simulink model "AutopilotControlSystem"  (R2021b)
settings: configuration reference "ctrlConfigSet" (kept outside this file)
undefined symbols (not defined in the file): ap, DiscIntNeverNeededParam, Earth, env, sensors, uavData, WGS84
libraries: mbdriLib x29, simulink x9, aerolibatmos2 x2, slpidlib x1, simulink_need_slupdate x1, aerolibconvert2 x1, aerolibtransform2 x1
(part 2 of 2)

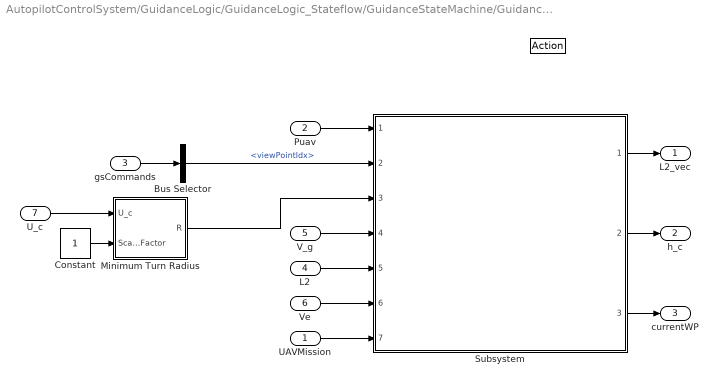
== system AutopilotControlSystem/GuidanceLogic/GuidanceLogic_Stateflow/GuidanceStateMachine/GuidanceLogic.Orbit ==
  UAVMission : Inport
  Puav : Inport  Port=2
  gsCommands : Inport  Port=3
  L2 : Inport  Port=4
  V_g : Inport  Port=5
  Ve : Inport  Port=6
  U_c : Inport  Port=7
  " " : ActionPort
      settings: CopyFcn=Stateflow.SLINSF.SimulinkMan.removeBlockPreDeleteFcn  PreDeleteFcn=Stateflow.SLINSF.SimulinkMan.unsafePredeleteFcn
  Bus Selector : BusSelector  OutputSignals=viewPointIdx
  Constant : Constant  OutDataTypeStr=single
      settings: AttributesFormatString=%<Value>
  Minimum Turn Radius : Subsystem
  Subsystem : Subsystem  ReferencedSubsystem=Orbit
  L2_vec : Outport  VectorParamsAs1DForOutWhenUnconnected=off
  h_c : Outport  Port=2  VectorParamsAs1DForOutWhenUnconnected=off
  currentWP : Outport  Port=3  VectorParamsAs1DForOutWhenUnconnected=off
  wires:
  Subsystem/2 -> h_c/1
  Subsystem/3 -> currentWP/1
  Subsystem/1 -> L2_vec/1
  UAVMission/1 -> Subsystem/7
  Puav/1 -> Subsystem/1
  gsCommands/1 -> Bus Selector/1
  Bus Selector/1 -> Subsystem/2  "<viewPointIdx>"
  Constant/1 -> Minimum Turn Radius/2(Scale Factor)
  U_c/1 -> Minimum Turn Radius/1(U_c)
  Minimum Turn Radius/1(R) -> Subsystem/3
  L2/1 -> Subsystem/5
  V_g/1 -> Subsystem/4
  Ve/1 -> Subsystem/6

== system AutopilotControlSystem/GuidanceLogic/GuidanceLogic_Stateflow/GuidanceStateMachine/GuidanceLogic.RTB ==
  gsCommands : Inport  OutDataTypeStr=Bus: gsCommandsBus
  UAVMission : Inport  Port=2
  Puav : Inport  Port=3
  " " : ActionPort
      settings: CopyFcn=Stateflow.SLINSF.SimulinkMan.removeBlockPreDeleteFcn  PreDeleteFcn=Stateflow.SLINSF.SimulinkMan.unsafePredeleteFcn
  Bus Selector : BusSelector  OutputSignals=MobileLocation,followMobile,h_c_midLevel
  Subsystem : Subsystem  ReferencedSubsystem=RTB_FollowMobile
  L2_vec : Outport  VectorParamsAs1DForOutWhenUnconnected=off
  h_c : Outport  Port=2  VectorParamsAs1DForOutWhenUnconnected=off
  currentWP : Outport  Port=3  VectorParamsAs1DForOutWhenUnconnected=off
  wires:
  Subsystem/2 -> h_c/1
  Subsystem/1 -> L2_vec/1
  Subsystem/3 -> currentWP/1
  Puav/1 -> Subsystem/4
  UAVMission/1 -> Subsystem/5
  gsCommands/1 -> Bus Selector/1
  Bus Selector/1 -> Subsystem/1  "<MobileLocation>"
  Bus Selector/2 -> Subsystem/2  "<followMobile>"
  Bus Selector/3 -> Subsystem/3  "<h_c_midLevel>"

== system AutopilotControlSystem/GuidanceLogic/GuidanceLogic_Stateflow/GuidanceStateMachine/GuidanceLogic.WP ==
  apConfigParams : Inport
  UAVMission : Inport  Port=2
  Puav : Inport  Port=3
  L2 : Inport  Port=4
  V_g : Inport  Port=5
  wpEnable : Inport  Port=6
  " " : ActionPort
      settings: CopyFcn=Stateflow.SLINSF.SimulinkMan.removeBlockPreDeleteFcn  PreDeleteFcn=Stateflow.SLINSF.SimulinkMan.unsafePredeleteFcn
  Bus Selector : BusSelector  OutputSignals=turnLead
  MATLAB Function : MATLAB Function  TreatAsAtomicUnit=on
  Subsystem Reference : Subsystem  ReferencedSubsystem=WP_Guidance
  L2_vec : Outport  VectorParamsAs1DForOutWhenUnconnected=off
  h_c : Outport  Port=2  VectorParamsAs1DForOutWhenUnconnected=off
  currentWP : Outport  Port=3  VectorParamsAs1DForOutWhenUnconnected=off
  wires:
  UAVMission/1 -> MATLAB Function/1(u), Subsystem Reference/1
  Subsystem Reference/3 -> currentWP/1
  Subsystem Reference/2 -> h_c/1
  Subsystem Reference/1 -> L2_vec/1
  Puav/1 -> Subsystem Reference/2
  L2/1 -> Subsystem Reference/3
  MATLAB Function/1(maxWp) -> Subsystem Reference/4
  apConfigParams/1 -> Bus Selector/1
  Bus Selector/1 -> Subsystem Reference/5  "<turnLead>"
  V_g/1 -> Subsystem Reference/6
  wpEnable/1 -> Subsystem Reference/7

== system AutopilotControlSystem/GuidanceLogic/GuidanceLogic_Stateflow/Recent Enable ==
  WP Fly : Inport
  IC1 : InitialCondition  Value=0
  Subsystem : Subsystem
  WPEnable : Outport  VectorParamsAs1DForOutWhenUnconnected=off
  wires:
  WP Fly/1 -> IC1/1
  Subsystem/1(Just Enab) -> WPEnable/1
  IC1/1 -> Subsystem/1(WP Fly)

== system AutopilotControlSystem/InnerLoopAutopilot/Latch Trim Conditions/Latch Control Surfaces Trim from any mode ==
  ctrlSurfaces : Inport
  Trigger : TriggerPort  TriggerType=falling  VariantControl=Variant
  Trim : Outport  VectorParamsAs1DForOutWhenUnconnected=off
  wires:
  ctrlSurfaces/1 -> Trim/1

== system AutopilotControlSystem/InnerLoopAutopilot/Longitudinal Channel/Compute Feed Forward ==
  dEFFGain : Inport
  SensorData : Inport  Port=2
  1D Discrete Filter : mbdriLib/Filtering/1D Discrete Filter  bw=10  TSample=ap.apSampleTime
      settings: AttributesFormatString=Fc = 10
  Add5 : Sum  Inputs=+-  OutDataTypeStr=single
  Bus Selector : BusSelector  OutputSignals=Euler
  Constant2 : Constant  OutDataTypeStr=single
      settings: AttributesFormatString=%<Value>
  Constant4 : Constant  OutDataTypeStr=single
      settings: AttributesFormatString=%<Value>
  Product : Product  Inputs=*/  RndMeth=Zero
  Product1 : Product  RndMeth=Zero
  Selector : Selector  InputPortWidth=3  IndexOptions=Index vector (dialog)  Indices=[1]  OutputSizes=1
  Trigonometric Function : Trigonometry  Operator=cos
  "[-60 60]" : Saturate  UpperLimit=60  LowerLimit=-60
      settings: AttributesFormatString="[%<LowerLimit>  %<UpperLimit>]"
  FF : Outport  VectorParamsAs1DForOutWhenUnconnected=off
  wires:
  Selector/1 -> 1D Discrete Filter/1
  Product/1 -> Add5/1
  Constant4/1 -> Product/1
  1D Discrete Filter/1 -> "[-60 60]"/1
  Trigonometric Function/1 -> Product/2
  Constant2/1 -> Add5/2
  Product1/1 -> FF/1
  Add5/1 -> Product1/2
  "[-60 60]"/1 -> Trigonometric Function/1
  Bus Selector/1 -> Selector/1  "<Euler>"
  dEFFGain/1 -> Product1/1
  SensorData/1 -> Bus Selector/1

== system AutopilotControlSystem/InnerLoopAutopilot/Longitudinal Channel/Height Error to Pitch Command [PI] ==
  Error : Inport
  Reset : Inport  Port=2
  PIDGains : Inport  Port=3
  Cast To Boolean : DataTypeConversion  OutDataTypeStr=boolean
  Demux : Demux  Outputs=3
  PID Controller : slpidlib/PID Controller  Controller=PI  Form=Parallel  TimeDomain=Discrete-time  UseExternalTs=off  SampleTime=ap.apSampleTime  IntegratorMethod=Trapezoidal  FilterMethod=Forward Euler  ControllerParametersSource=external  P=1  I=1  D=0  UseFilter=on  N=100  TunerSelectOption=Transfer Function Based (PID Tuner App)  InitialConditionSource=internal  InitialConditionForIntegrator=0  InitialConditionForFilter=0  DifferentiatorICPrevScaledInput=0  ExternalReset=level  TrackingMode=off  Kt=1  LimitOutput=on  SatLimitsSource=internal  UpperSaturationLimit=ap.control.the_cLimit  LowerSaturationLimit=-ap.control.the_cLimit  LinearizeAsGain=on  AntiWindupMode=clamping  Kb=1  POutMin=[]  POutMax=[]  IOutMin=[]  IOutMax=[]  DOutMin=[]  DOutMax=[]  NOutMin=[]  NOutMax=[]  SumOutMin=[]  SumOutMax=[]  SaturationOutMin=[]  SaturationOutMax=[]  PParamMin=[]  PParamMax=[]  IParamMin=[]  IParamMax=[]  DParamMin=[]  DParamMax=[]  NParamMin=[]  NParamMax=[]  KbParamMin=[]  KbParamMax=[]  KtParamMin=[]  KtParamMax=[]  KbOutMin=[]  KbOutMax=[]  KtOutMin=[]  KtOutMax=[]  IntegratorOutMin=[]  IntegratorOutMax=[]  FilterOutMin=[]  FilterOutMax=[]  SumI1OutMin=[]  SumI1OutMax=[]  SumI2OutMin=[]  SumI2OutMax=[]  SumI3OutMin=[]  SumI3OutMax=[]  SumI4OutMin=[]  SumI4OutMax=[]  SumDOutMin=[]  SumDOutMax=[]  DifferentiatorOutMin=[]  DifferentiatorOutMax=[]  FilterDiffOutCoefMin=[]  FilterDiffOutCoefMax=[]  ReciprocalOutMin=[]  ReciprocalOutMax=[]  SumDenOutMin=[]  SumDenOutMax=[]  SumNumOutMin=[]  SumNumOutMax=[]  DivideOutMin=[]  DivideOutMax=[]  UdiffTsProdOutMin=[]  UdiffTsProdOutMax=[]  NTsProdOutMin=[]  NTsProdOutMax=[]  UintegralTsProdOutMin=[]  UintegralTsProdOutMax=[]  UngainTsProdOutMin=[]  UngainTsProdOutMax=[]  IntegratorContinuousStateAttributes=''  IntegratorStateMustResolveToSignalObject=off  IntegratorRTWStateStorageClass=Auto  FilterContinuousStateAttributes=''  FilterStateMustResolveToSignalObject=off  FilterRTWStateStorageClass=Auto  ParallelPVariant=ExternalParameters  IdealPVariant=Disabled  IVariant=ExternalParameters  DVariant=Disabled  IntegratorVariant=Discrete  SatVariant=Enabled  AWVariant=DiscClampingParallel  PCopyVariant=Disabled  TRVariant=Disabled  FdbkBlocksVariant=Feedback  IdealPFdbkVariant=Passthrough  SatFdbkVariant=Passthrough  DerivativeFilterVariant=Disabled  NVariant=Disabled  NCopyVariant=Disabled_SignalSpec  FilterICVariant=Disabled  IntegratorICVariant=InternalICs  ExternalResetVariant=ExternalReset  TRSumVariant=Passthrough  SumFdbkVariant=Enabled  SumVariant=Sum_PI  TsampFilterVariant=InternalTs  TsampNgainVariant=Passthrough  TsampIntegralVariant=Passthrough  ExternalSaturationOutDataTypeStr=Inherit: Same as second input
  Terminator : Terminator
  Output : Outport  VectorParamsAs1DForOutWhenUnconnected=off
  wires:
  Demux/3 -> Terminator/1
  Error/1 -> PID Controller/1
  PIDGains/1 -> Demux/1
  Demux/1 -> PID Controller/2
  Demux/2 -> PID Controller/3
  Reset/1 -> Cast To Boolean/1
  PID Controller/1 -> Output/1
  Cast To Boolean/1 -> PID Controller/4

== system AutopilotControlSystem/InnerLoopAutopilot/Longitudinal Channel/Rate Limiter Dynamic with External IC and Autoreset for Change in IC ==
  note: Y(k)
  note: U(k)
  up : Inport
  u : Inport  Port=2
  IC : Inport  Port=3
  lo : Inport  Port=4
  Capture/Reset IC : Subsystem
  Difference Inputs1 : Sum  Description=Add in CPU  DisableCoverage=on  Inputs=+-  OutDataTypeStr=Inherit: Inherit via back propagation
  Difference Inputs2 : Sum  Description=Add in CPU  OutDataTypeStr=Inherit: Inherit via back propagation
  FixPt Data Type Duplicate : DataTypeDuplicate  DisableCoverage=on  NumInputPorts=7
  Saturation Dynamic : simulink/Discontinuities/Saturation Dynamic  OutMin=[]  OutMax=[]  OutDataTypeStr=Inherit: Same as second input  OutDataType=fixdt(1, 16)  OutScaling=2^-10  DoSatur=off
  delta fall limit : Product  DisableCoverage=on  Inputs=**  OutDataTypeStr=Inherit: Inherit via back propagation  SaturateOnIntegerOverflow=on
  delta rise limit : Product  DisableCoverage=on  Inputs=**  OutDataTypeStr=Inherit: Inherit via back propagation  SaturateOnIntegerOverflow=on
  sample time : SampleTimeMath  DisableCoverage=on  TsampMathOp=Ts Only  weightValue=1
  Y : Outport  VectorParamsAs1DForOutWhenUnconnected=off
  wires:
  sample time/1 -> delta fall limit/2, delta rise limit/2
  lo/1 -> delta fall limit/1
  delta rise limit/1 -> FixPt Data Type Duplicate/6, Saturation Dynamic/1
  up/1 -> delta rise limit/1
  Difference Inputs2/1 -> FixPt Data Type Duplicate/1, Capture/Reset IC/1(Y(k)), Y/1
  Saturation Dynamic/1 -> Difference Inputs2/1, FixPt Data Type Duplicate/7
  delta fall limit/1 -> FixPt Data Type Duplicate/3, Saturation Dynamic/3
  u/1 -> Difference Inputs1/1, FixPt Data Type Duplicate/5, sample time/1
  Difference Inputs1/1 -> FixPt Data Type Duplicate/4, Saturation Dynamic/2  "( U(k) - Y(k-1) )"
  Capture/Reset IC/1(Y(k-1)) -> Difference Inputs2/2, FixPt Data Type Duplicate/2, Difference Inputs1/2
  IC/1 -> Capture/Reset IC/2(IC)

== system AutopilotControlSystem/Navigation Filter/Get Vn Ve/Subsystem5 ==
  u : Inport
  Trigonometric Function : Trigonometry
  Trigonometric Function1 : Trigonometry  Operator=cos
  sin(u) : Outport  VectorParamsAs1DForOutWhenUnconnected=off
  cos(u) : Outport  Port=2  VectorParamsAs1DForOutWhenUnconnected=off
  wires:
  u/1 -> Trigonometric Function/1, Trigonometric Function1/1
  Trigonometric Function/1 -> sin(u)/1
  Trigonometric Function1/1 -> cos(u)/1

== system AutopilotControlSystem/Navigation Filter/Position&Velocity Filter/CompRateOnly ==
  LoPass : Inport
  Gain : Gain  Gain=omega
      settings: AttributesFormatString=%<Gain>
  Sum1 : Sum  Inputs=|+-
  Unit Delay : UnitDelay  SampleTime=T  HasFrameUpgradeWarning=on
  ZPK 1D Discrete Filter : mbdriLib/Filtering/ZPK 1D Discrete Filter  zval=[]  pval=[0]  kval=1  TSample=0.01
  Rate_hat : Outport  VectorParamsAs1DForOutWhenUnconnected=off
  wires:
  Unit Delay/1 -> Sum1/2
  LoPass/1 -> Sum1/1
  Sum1/1 -> Gain/1
  Gain/1 -> ZPK 1D Discrete Filter/1, Rate_hat/1
  ZPK 1D Discrete Filter/1 -> Unit Delay/1

== system AutopilotControlSystem/Navigation Filter/Position&Velocity Filter/Deriv  ==
  y : Inport
  Gain2 : Gain  Gain=[ 1/(5*ap.apSampleTime) ]
      settings: AttributesFormatString=%<Gain>
  Integer Delay1 : Delay  DelayLength=5  InitialCondition=0
  Sum5 : Sum  Inputs=-+|
  ydot : Outport  VectorParamsAs1DForOutWhenUnconnected=off
  wires:
  Gain2/1 -> ydot/1
  y/1 -> Integer Delay1/1, Sum5/2
  Integer Delay1/1 -> Sum5/1
  Sum5/1 -> Gain2/1

== system AutopilotControlSystem/Navigation Filter/Position&Velocity Filter/VN Ve Filter ==
  Vn : Inport
  Ve : Inport  Port=2
  New GPS : Inport  Port=3
  Enable : EnablePort
  Constant : Constant  Value=ap.apSampleTime
      settings: AttributesFormatString=%<Value>
  RateAid for GPS : mbdriLib/Filtering/RateAid for GPS  SystemSampleTime=-1  VariantActivationTime=update diagram  Latency=0  AutoFrameSizeCalculation=off
  RateAid for GPS1 : mbdriLib/Filtering/RateAid for GPS  SystemSampleTime=-1  VariantActivationTime=update diagram  Latency=0  AutoFrameSizeCalculation=off
  Vn_fil : Outport  OutputWhenDisabled=reset  InitialOutput=0  VectorParamsAs1DForOutWhenUnconnected=off
  Ve_fil : Outport  Port=2  OutputWhenDisabled=reset  InitialOutput=0  VectorParamsAs1DForOutWhenUnconnected=off
  wires:
  Constant/1 -> RateAid for GPS1/3, RateAid for GPS/3
  New GPS/1 -> RateAid for GPS/2, RateAid for GPS1/2
  Vn/1 -> RateAid for GPS/1
  Ve/1 -> RateAid for GPS1/1
  RateAid for GPS/1 -> Vn_fil/1
  RateAid for GPS1/1 -> Ve_fil/1

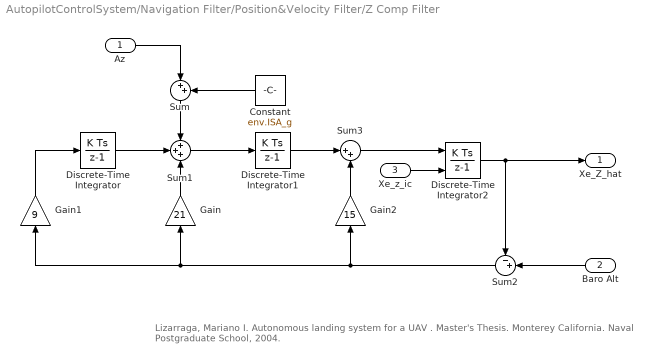
== system AutopilotControlSystem/Navigation Filter/Position&Velocity Filter/Z Comp Filter ==
  note: Lizarraga, Mariano I. Autonomous landing system for a UAV . Master's Thesis. Monterey California. Naval Postgraduate School, 2004.
  Az : Inport
  Baro Alt : Inport  Port=2
  Xe_z_ic : Inport  Port=3
  Constant : Constant  Value=env.ISA_g
      settings: AttributesFormatString=%<Value>
  Discrete-Time Integrator : DiscreteIntegrator  gainval=1  SampleTime=-1  ICPrevOutput=DiscIntNeverNeededParam  ICPrevScaledInput=DiscIntNeverNeededParam
  Discrete-Time Integrator1 : DiscreteIntegrator  gainval=1  SampleTime=-1  ICPrevOutput=DiscIntNeverNeededParam  ICPrevScaledInput=DiscIntNeverNeededParam
  Discrete-Time Integrator2 : DiscreteIntegrator  gainval=1  InitialConditionSource=external  SampleTime=-1  ICPrevOutput=DiscIntNeverNeededParam  ICPrevScaledInput=DiscIntNeverNeededParam
  Gain : Gain  Gain=21  OutDataTypeStr=single
      settings: AttributesFormatString=%<Gain>
  Gain1 : Gain  Gain=9  OutDataTypeStr=single
      settings: AttributesFormatString=%<Gain>
  Gain2 : Gain  Gain=15  OutDataTypeStr=single
      settings: AttributesFormatString=%<Gain>
  Sum : Sum  Inputs=|++
  Sum1 : Sum  Inputs=+++
  Sum2 : Sum  Inputs=-+|
  Sum3 : Sum  Inputs=|++
  Xe_Z_hat : Outport  VectorParamsAs1DForOutWhenUnconnected=off
  wires:
  Discrete-Time Integrator2/1 -> Sum2/1, Xe_Z_hat/1
  Gain2/1 -> Sum3/2
  Gain1/1 -> Discrete-Time Integrator/1
  Gain/1 -> Sum1/3
  Sum2/1 -> Gain2/1, Gain/1, Gain1/1
  Sum3/1 -> Discrete-Time Integrator2/1
  Discrete-Time Integrator1/1 -> Sum3/1
  Baro Alt/1 -> Sum2/2
  Xe_z_ic/1 -> Discrete-Time Integrator2/2
  Sum1/1 -> Discrete-Time Integrator1/1
  Sum/1 -> Sum1/1
  Discrete-Time Integrator/1 -> Sum1/2
  Constant/1 -> Sum/2
  Az/1 -> Sum/1

== system AutopilotControlSystem/GuidanceLogic/GuidanceLogic_Simulink/Determine RTB/getHeartbeatAge ==
  Heartbeat : Inport
  Constant : Constant
  Discrete-Time Integrator : DiscreteIntegrator  ExternalReset=level  SampleTime=-1  LimitOutput=on  UpperSaturationLimit=50  LowerSaturationLimit=0  ICPrevOutput=DiscIntNeverNeededParam  ICPrevScaledInput=DiscIntNeverNeededParam
  Age : Outport  VectorParamsAs1DForOutWhenUnconnected=off
  wires:
  Heartbeat/1 -> Discrete-Time Integrator/2
  Discrete-Time Integrator/1 -> Age/1
  Constant/1 -> Discrete-Time Integrator/1

== system AutopilotControlSystem/GuidanceLogic/GuidanceLogic_Simulink/Guidance/Circle Guidance ==
  Xe : Inport
  InterestPoint : Inport  Port=2
  R : Inport  Port=3
  |V_g| : Inport  Port=4
  L2 : Inport  Port=5
  Ve : Inport  Port=6
  UAVMission : Inport  Port=7
  Action Port : ActionPort  ActionPortLabel=elseif( u1 == 3)
  Subsystem : Subsystem  ReferencedSubsystem=Orbit
  L2_vec : Outport  VectorParamsAs1DForOutWhenUnconnected=off
  h_c : Outport  Port=2  VectorParamsAs1DForOutWhenUnconnected=off
  currentWP : Outport  Port=3  VectorParamsAs1DForOutWhenUnconnected=off
  wires:
  |V_g|/1 -> Subsystem/4
  Subsystem/1 -> L2_vec/1
  Subsystem/3 -> currentWP/1
  Subsystem/2 -> h_c/1
  UAVMission/1 -> Subsystem/7
  Ve/1 -> Subsystem/6
  L2/1 -> Subsystem/5
  R/1 -> Subsystem/3
  InterestPoint/1 -> Subsystem/2
  Xe/1 -> Subsystem/1

== system AutopilotControlSystem/GuidanceLogic/GuidanceLogic_Simulink/Guidance/Mid Level Direct Commands ==
  psiDot_c_ml : Inport
  h_c_midLvl : Inport  Port=2
  U_m : Inport  Port=3
  Action Port : ActionPort  ActionPortLabel=elseif( u1 == 4)
  Subsystem : Subsystem  ReferencedSubsystem=DirectCommands
  phi_c_ml : Outport  VectorParamsAs1DForOutWhenUnconnected=off
  h_c : Outport  Port=2  VectorParamsAs1DForOutWhenUnconnected=off
  currentWP : Outport  Port=3  VectorParamsAs1DForOutWhenUnconnected=off
  wires:
  Subsystem/3 -> currentWP/1
  Subsystem/2 -> h_c/1
  Subsystem/1 -> phi_c_ml/1
  U_m/1 -> Subsystem/3
  psiDot_c_ml/1 -> Subsystem/1
  h_c_midLvl/1 -> Subsystem/2

== system AutopilotControlSystem/GuidanceLogic/GuidanceLogic_Simulink/Guidance/Minimum Turn Radius ==
  U_c : Inport
  Scale Factor : Inport  Port=2
  Constant1 : Constant  Value=ap.guidance.maxAcc
      settings: AttributesFormatString=%<Value>
  IC : InitialCondition  Value=1.5
  Math Function : Math  Operator=square  SignedPower=on  SaturateOnIntegerOverflow=on
  Product2 : Product  RndMeth=Zero
  Product3 : Product  Inputs=*/  RndMeth=Zero
  "[1.5 10]" : Saturate  UpperLimit=10  LowerLimit=1.5
      settings: AttributesFormatString="[%<LowerLimit>  %<UpperLimit>]"
  R : Outport  VectorParamsAs1DForOutWhenUnconnected=off
  wires:
  IC/1 -> "[1.5 10]"/1
  "[1.5 10]"/1 -> Product2/1
  Product3/1 -> R/1
  Scale Factor/1 -> IC/1
  Math Function/1 -> Product2/2
  Constant1/1 -> Product3/2
  Product2/1 -> Product3/1
  U_c/1 -> Math Function/1

== system AutopilotControlSystem/GuidanceLogic/GuidanceLogic_Simulink/Guidance/RTB//Follow Mobile Guidance ==
  Mobile Location : Inport
  Follow Mobile? : Inport  Port=2
  MidLvl h_c : Inport  Port=3
  Puav : Inport  Port=4
  UAVMission : Inport  Port=5
  Action Port : ActionPort  ActionPortLabel=if(u2 == 1)
  Subsystem : Subsystem  ReferencedSubsystem=RTB_FollowMobile
  L2_vec : Outport  VectorParamsAs1DForOutWhenUnconnected=off
  h_c : Outport  Port=2  VectorParamsAs1DForOutWhenUnconnected=off
  currentWP : Outport  Port=3  VectorParamsAs1DForOutWhenUnconnected=off
  wires:
  Mobile Location/1 -> Subsystem/1
  Follow Mobile?/1 -> Subsystem/2
  MidLvl h_c/1 -> Subsystem/3
  Puav/1 -> Subsystem/4
  UAVMission/1 -> Subsystem/5
  Subsystem/1 -> L2_vec/1
  Subsystem/2 -> h_c/1
  Subsystem/3 -> currentWP/1

== system AutopilotControlSystem/GuidanceLogic/GuidanceLogic_Simulink/Guidance/Recent Enable ==
  WP Fly : Inport
  IC1 : InitialCondition  Value=0
  Subsystem : Subsystem
  WPEnable : Outport  VectorParamsAs1DForOutWhenUnconnected=off
  wires:
  WP Fly/1 -> IC1/1
  Subsystem/1(Just Enab) -> WPEnable/1
  IC1/1 -> Subsystem/1(WP Fly)

== system AutopilotControlSystem/GuidanceLogic/GuidanceLogic_Simulink/Guidance/WP Guidance ==
  UAVMission : Inport
  Xe : Inport  Port=2
  L2 : Inport  Port=3
  MaxWP : Inport  Port=4
  turnLeadTime : Inport  Port=5
  V_g : Inport  Port=6
  WpEnable : Inport  Port=7
  Action Port : ActionPort  ActionPortLabel=elseif(u1 == 2)
  Subsystem Reference : Subsystem  ReferencedSubsystem=WP_Guidance
  L2Vec : Outport  VectorParamsAs1DForOutWhenUnconnected=off
  h_c : Outport  Port=2  VectorParamsAs1DForOutWhenUnconnected=off
  currentWP : Outport  Port=3  VectorParamsAs1DForOutWhenUnconnected=off
  wires:
  Subsystem Reference/1 -> L2Vec/1
  Subsystem Reference/2 -> h_c/1
  Subsystem Reference/3 -> currentWP/1
  UAVMission/1 -> Subsystem Reference/1
  Xe/1 -> Subsystem Reference/2
  L2/1 -> Subsystem Reference/3
  MaxWP/1 -> Subsystem Reference/4
  turnLeadTime/1 -> Subsystem Reference/5
  V_g/1 -> Subsystem Reference/6
  WpEnable/1 -> Subsystem Reference/7

== system AutopilotControlSystem/GuidanceLogic/GuidanceLogic_Stateflow/Determine RTB/getHeartbeatAge ==
  Heartbeat : Inport
  Constant : Constant
  Discrete-Time Integrator : DiscreteIntegrator  ExternalReset=level  SampleTime=-1  LimitOutput=on  UpperSaturationLimit=50  LowerSaturationLimit=0  ICPrevOutput=DiscIntNeverNeededParam  ICPrevScaledInput=DiscIntNeverNeededParam
  Age : Outport  VectorParamsAs1DForOutWhenUnconnected=off
  wires:
  Heartbeat/1 -> Discrete-Time Integrator/2
  Discrete-Time Integrator/1 -> Age/1
  Constant/1 -> Discrete-Time Integrator/1

== system AutopilotControlSystem/GuidanceLogic/GuidanceLogic_Stateflow/GuidanceStateMachine/GuidanceLogic.Orbit/Minimum Turn Radius ==
  U_c : Inport
  Scale Factor : Inport  Port=2
  Constant1 : Constant  Value=ap.guidance.maxAcc
      settings: AttributesFormatString=%<Value>
  IC : InitialCondition  Value=1.5
  Math Function : Math  Operator=square  SignedPower=on  SaturateOnIntegerOverflow=on
  Product2 : Product  RndMeth=Zero
  Product3 : Product  Inputs=*/  RndMeth=Zero
  "[1.5 10]" : Saturate  UpperLimit=10  LowerLimit=1.5
      settings: AttributesFormatString="[%<LowerLimit>  %<UpperLimit>]"
  R : Outport  VectorParamsAs1DForOutWhenUnconnected=off
  wires:
  IC/1 -> "[1.5 10]"/1
  "[1.5 10]"/1 -> Product2/1
  Product3/1 -> R/1
  Scale Factor/1 -> IC/1
  Math Function/1 -> Product2/2
  Constant1/1 -> Product3/2
  Product2/1 -> Product3/1
  U_c/1 -> Math Function/1

== system AutopilotControlSystem/GuidanceLogic/GuidanceLogic_Stateflow/Recent Enable/Subsystem ==
  WP Fly : Inport
  Data Type Conversion1 : DataTypeConversion  OutDataTypeStr=double
  Data Type Conversion2 : DataTypeConversion  OutDataTypeStr=uint8
  Hit Crossing : HitCross  HitCrossingOffset=0.5  HitCrossingDirection=rising
  Just Enab : Outport  VectorParamsAs1DForOutWhenUnconnected=off
  wires:
  Data Type Conversion1/1 -> Hit Crossing/1
  Hit Crossing/1 -> Data Type Conversion2/1
  Data Type Conversion2/1 -> Just Enab/1
  WP Fly/1 -> Data Type Conversion1/1

== system AutopilotControlSystem/InnerLoopAutopilot/Longitudinal Channel/Rate Limiter Dynamic with External IC and Autoreset for Change in IC/Capture//Reset IC ==
  Y(k) : Inport
  IC : Inport  Port=2
  Abs : Abs
  Delay : Delay  DelayLength=1
  Subsystem : Subsystem
  Subtract : Sum  Inputs=+-
  Unit Delay Resettable External IC : simulink_need_slupdate/Unit Delay Resettable External IC  tsamp=-1
      settings: SourceProductBaseCode=SL
  Y(k-1) : Outport  VectorParamsAs1DForOutWhenUnconnected=off
  wires:
  Unit Delay Resettable External IC/1 -> Y(k-1)/1  "Y(k-1)"
  Y(k)/1 -> Unit Delay Resettable External IC/1
  Subtract/1 -> Abs/1
  Abs/1 -> Subsystem/1(WP Fly)
  IC/1 -> Delay/1, Subtract/2, Unit Delay Resettable External IC/3
  Subsystem/1(Just Enab) -> Unit Delay Resettable External IC/2
  Delay/1 -> Subtract/1

== system AutopilotControlSystem/GuidanceLogic/GuidanceLogic_Simulink/Guidance/Recent Enable/Subsystem ==
  WP Fly : Inport
  Data Type Conversion1 : DataTypeConversion  OutDataTypeStr=double
  Data Type Conversion2 : DataTypeConversion  OutDataTypeStr=uint8
  Hit Crossing : HitCross  HitCrossingOffset=0.5  HitCrossingDirection=rising
  Just Enab : Outport  VectorParamsAs1DForOutWhenUnconnected=off
  wires:
  Data Type Conversion1/1 -> Hit Crossing/1
  Hit Crossing/1 -> Data Type Conversion2/1
  Data Type Conversion2/1 -> Just Enab/1
  WP Fly/1 -> Data Type Conversion1/1

== system AutopilotControlSystem/InnerLoopAutopilot/Longitudinal Channel/Rate Limiter Dynamic with External IC and Autoreset for Change in IC/Capture//Reset IC/Subsystem ==
  WP Fly : Inport
  Compare To Constant : simulink/Logic and Bit Operations/Compare To Constant  relop=>=  const=0.5  OutDataTypeStr=boolean
  Compare To Constant1 : simulink/Logic and Bit Operations/Compare To Constant  relop=<  const=0.5  OutDataTypeStr=boolean
  Logical Operator : Logic  AllPortsSameDT=off  OutDataTypeStr=boolean
  Unit Delay : UnitDelay  SampleTime=-1  HasFrameUpgradeWarning=on
  Just Enab : Outport  VectorParamsAs1DForOutWhenUnconnected=off
  wires:
  WP Fly/1 -> Unit Delay/1, Compare To Constant/1
  Compare To Constant/1 -> Logical Operator/1
  Compare To Constant1/1 -> Logical Operator/2
  Unit Delay/1 -> Compare To Constant1/1
  Logical Operator/1 -> Just Enab/1

== matlab function AutopilotControlSystem/GuidanceLogic/GuidanceLogic_Stateflow/GuidanceStateMachine/GuidanceLogic.WP/MATLAB Function ==
  data: u input Bus: waypoint size=10; maxWp output
function maxWp = getMaxWp(u)
%#codegen

for ii=1:10
    wp = u(ii);
    if wp.wpPos(1) == 0
        maxWp = uint8(ii-1);
        return 
    end
end

maxWp = uint8(10);

== stateflow chart AutopilotControlSystem/GuidanceLogic/GuidanceLogic_Stateflow/GuidanceStateMachine ==
  settings: updateMethod=DISCRETE  sampleTime=ap.apSampleTime
  state GuidanceLogic
    state RTB
    state WP
    state Orbit
    state MidLevel
    (default) -> (junction 43)
    (junction 83) -> RTB
    (junction 82) -> (junction 83)
    (junction 43) -> RTB [order 1] : [RTB==1]
    (junction 43) -> (junction 19) [order 2]
    (junction 19) -> WP [order 1] : [guidanceMode == 2]
    (junction 19) -> (junction 27) [order 2]
    (junction 27) -> Orbit [order 1] : [guidanceMode == 3]
    (junction 27) -> (junction 32) [order 2]
    (junction 32) -> MidLevel [order 1] : [guidanceMode == 4]
    (junction 32) -> (junction 84) [order 2]
    (junction 84) -> (junction 82)
  (default) -> GuidanceLogic
  GuidanceLogic -> GuidanceLogic : [hasChanged(RTB) || hasChanged(guidanceMode)]
  data: sf_internal_action_state_placeholder_data local double size=1 =0; sf_internal_action_state_placeholder_data local double size=1 =0; sf_internal_action_state_placeholder_data local double size=1 =0; sf_internal_action_state_placeholder_data local double size=1 =0; gsCommands input; currentWP output; h_c output; phi_c_ml output; L2_vec output; UAVMission input; apConfigParams input; Puav input; L2 input; V_g input; wpEnable input; U_c input; Ve input; guidanceMode input; RTB input

== matlab function AutopilotControlSystem/GuidanceLogic/GuidanceLogic_Simulink/MATLAB Function ==
  data: u input Bus: waypoint size=10; maxWp output
function maxWp = getMaxWp(u)
%#codegen

for ii=1:10
    wp = u(ii);
    if wp.wpPos(1) == 0
        maxWp = uint8(ii-1);
        return 
    end
end

maxWp = uint8(10);
